simulink subsystem "SD_Filter"  (R2022b)
settings: Solver=VariableStepAuto  StartTime=0.0  StopTime=10.0  RelTol=1e-3
undefined symbols (not defined in the file or in its folder): bitwidths
settings Model: Creator=1111293  LastModifiedBy=qaztr
settings SolverCC: AlgebraicLoopSolver=TrustRegion
settings DebuggingCC: UnconnectedInputMsg=warning  UnconnectedOutputMsg=warning  UnconnectedLineMsg=warning  SFMachineParentedDataDiag=warning
settings ModelReferenceCC: EnableRefExpFcnMdlSchedulingChecks=on
settings RTWCC: DLArmComputeVersion=19.05

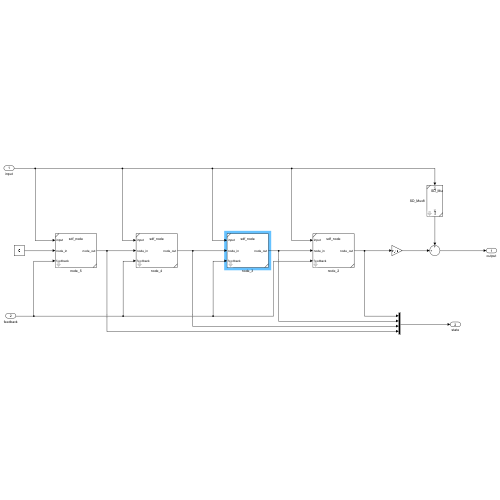
[thumbnail: Simulink's stored preview of the top-level diagram]
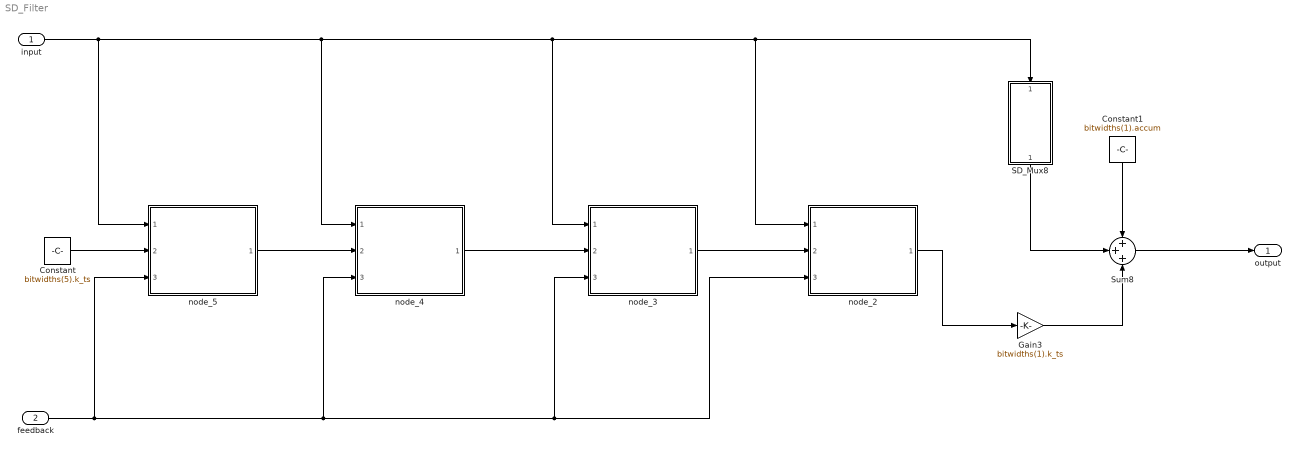
== system SD_Filter ==
  input : Inport
  feedback : Inport  Port=2
  Constant : Constant  Value=bitwidths(5).k_ts
  Constant1 : Constant  Value=bitwidths(1).accum
  Gain3 : Gain  Gain=bitwidths(1).k_ts  RndMeth=Round
  SD_Mux8 : Subsystem  ReferencedSubsystem=SD_Mux  a=bitwidths(1).beta  Parameter2=Inherit: Inherit via internal rule
  Sum8 : Sum  Inputs=+++  OutDataTypeStr=Inherit: Same as accumulator
  node_2 : Subsystem  ReferencedSubsystem=sdf_node  Parameter1=bitwidths(2).alpha  Parameter2=bitwidths(2).beta  Parameter3=bitwidths(2).k_ts  Parameter4=bitwidths(2).accum
  node_3 : Subsystem  ReferencedSubsystem=sdf_node  Parameter1=bitwidths(3).alpha  Parameter2=bitwidths(3).beta  Parameter3=bitwidths(3).k_ts  Parameter4=bitwidths(3).accum
  node_4 : Subsystem  ReferencedSubsystem=sdf_node  Parameter1=bitwidths(4).alpha  Parameter2=bitwidths(4).beta  Parameter3=bitwidths(4).k_ts  Parameter4=bitwidths(4).accum
  node_5 : Subsystem  ReferencedSubsystem=sdf_node  Parameter1=bitwidths(5).alpha  Parameter2=bitwidths(5).beta  Parameter3=bitwidths(5).k_ts  Parameter4=bitwidths(5).accum
  output : Outport
  wires:
  node_2/1 -> Gain3/1
  node_3/1 -> node_2/2
  node_4/1 -> node_3/2
  Sum8/1 -> output/1
  node_5/1 -> node_4/2
  feedback/1 -> node_3/3, node_2/3, node_4/3, node_5/3
  input/1 -> SD_Mux8/1, node_2/1, node_3/1, node_4/1, node_5/1
  Constant/1 -> node_5/2
  Gain3/1 -> Sum8/3
  SD_Mux8/1 -> Sum8/2
  Constant1/1 -> Sum8/1
